simulink model "TEST_ELEONORA"  (R2024b)
settings: Solver=ode4  StartTime=0.0  StopTime=simul.tf  FixedStep=0.01  RelTol=1e-3
undefined symbols (not defined in the file or in its folder): act, env, flag, IC, K, orb, sat, sens, ws
libraries: matrix_library x15, simulink_extras x5
(part 4 of 4)

== system TEST_ELEONORA/Real World/Hardware Models/Actuators/CMG + Control Logic/CMG/State/B assembler ==
  beta : Inport
  delta : Inport  Port=2
  Cos : Trigonometry  Operator=cos
  Cos1 : Trigonometry  Operator=cos
  Gain{,1..3} (4 alike) : Gain  Gain=-1
  Matrix Concatenate : Concatenate  NumInputs=4  Mode=Multidimensional array  ConcatenateDimension=2
  Matrix Concatenate{1..4} (4 alike) : Concatenate  NumInputs=3  Mode=Multidimensional array
  Product{,1..7} (8 alike) : Product
  Selector : Selector  InputPortWidth=4  IndexOptions=Index vector (dialog)  Indices=1  OutputSizes=1
  Selector1 : Selector  InputPortWidth=4  IndexOptions=Index vector (dialog)  Indices=1  OutputSizes=1
  Selector10 : Selector  InputPortWidth=4  IndexOptions=Index vector (dialog)  Indices=4  OutputSizes=1
  Selector11 : Selector  InputPortWidth=4  IndexOptions=Index vector (dialog)  Indices=4  OutputSizes=1
  Selector2 : Selector  InputPortWidth=4  IndexOptions=Index vector (dialog)  Indices=1  OutputSizes=1
  Selector3 : Selector  InputPortWidth=4  IndexOptions=Index vector (dialog)  Indices=2  OutputSizes=1
  Selector4 : Selector  InputPortWidth=4  IndexOptions=Index vector (dialog)  Indices=2  OutputSizes=1
  Selector5 : Selector  InputPortWidth=4  IndexOptions=Index vector (dialog)  Indices=2  OutputSizes=1
  Selector6 : Selector  InputPortWidth=4  IndexOptions=Index vector (dialog)  Indices=3  OutputSizes=1
  Selector7 : Selector  InputPortWidth=4  IndexOptions=Index vector (dialog)  Indices=3  OutputSizes=1
  Selector8 : Selector  InputPortWidth=4  IndexOptions=Index vector (dialog)  Indices=3  OutputSizes=1
  Selector9 : Selector  InputPortWidth=4  IndexOptions=Index vector (dialog)  Indices=4  OutputSizes=1
  Sin : Trigonometry
  Sin1 : Trigonometry
  B : Outport
  wires:
  Cos/1 -> [cosd]
  Sin/1 -> [sind]
  delta/1 -> Cos/1, Sin/1
  beta/1 -> Sin1/1, Cos1/1
  Sin1/1 -> [sinb]
  Cos1/1 -> [cosb]
  Gain/1 -> Matrix Concatenate1/1
  Gain1/1 -> Matrix Concatenate1/2
  Gain2/1 -> Matrix Concatenate2/2
  Gain3/1 -> Matrix Concatenate4/1
  Matrix Concatenate1/1 -> Matrix Concatenate/1
  Matrix Concatenate2/1 -> Matrix Concatenate/2
  Matrix Concatenate3/1 -> Matrix Concatenate/3
  Matrix Concatenate4/1 -> Matrix Concatenate/4
  Matrix Concatenate/1 -> B/1
  Product/1 -> Gain/1
  Product1/1 -> Matrix Concatenate1/3
  Product2/1 -> Gain2/1
  Product3/1 -> Matrix Concatenate2/3
  Product4/1 -> Matrix Concatenate3/1
  Product5/1 -> Matrix Concatenate3/3
  Product6/1 -> Matrix Concatenate4/2
  Product7/1 -> Matrix Concatenate4/3
  Selector/1 -> Gain1/1
  Selector1/1 -> Product1/2
  Selector2/1 -> Product/2
  Selector3/1 -> Matrix Concatenate2/1
  Selector4/1 -> Product2/1
  Selector5/1 -> Product3/2
  Selector6/1 -> Product5/2
  Selector7/1 -> Matrix Concatenate3/2
  Selector8/1 -> Product4/1
  Selector9/1 -> Gain3/1
  Selector10/1 -> Product6/2
  Selector11/1 -> Product7/2
  [sind] -> Selector/1
  [sind] -> Selector3/1
  [sind] -> Selector7/1
  [sind] -> Selector9/1
  [cosd] -> Selector2/1
  [cosd] -> Selector1/1
  [cosd] -> Selector5/1
  [cosd] -> Selector4/1
  [cosd] -> Selector8/1
  [cosd] -> Selector6/1
  [cosd] -> Selector11/1
  [cosd] -> Selector10/1
  [cosb] -> Product/1
  [cosb] -> Product2/2
  [cosb] -> Product4/2
  [cosb] -> Product6/1
  [sinb] -> Product1/1
  [sinb] -> Product3/1
  [sinb] -> Product5/1
  [sinb] -> Product7/1

== matlab function TEST_ELEONORA/Real World/Hardware Models/Actuators/CMG + Control Logic/MATLAB Function ==
  data: A input; y output; B input
function y = fcn(A, B)

y = mldivide(A,B);
